simulink model "model"  (Simulink 8.7)
settings: Solver=ode45  StartTime=0.0  StopTime=10.0  FixedStep=Ts  RelTol=1e-3
values from neighbouring files (symbols this model uses):
  Am = 1    [model_params.m]
  NP = 0.001    [model_params.m]
  R = 2    [model_params.m]
  to = round(rand * 100)    [model_params.m]
  Ts = 0.002    [model_params.m]
libraries: commanapbnd3 x2
settings Model: Creator=morozov  LastModifiedBy=morozov
settings DataIOCC: LimitDataPoints=off  SaveFormat=Dataset
settings DebuggingCC: UnderspecifiedInitializationDetection=Simplified  MergeDetectMultiDrivingBlocksExec=error
settings HardwareCC: ProdBitPerPointer=64  ProdLargestAtomicFloat=Float  ProdIntDivRoundTo=Zero  ProdEndianess=LittleEndian  ProdWordSize=64  ProdHWDeviceType=Intel->x86-64 (Windows64)
settings ModelReferenceCC: PropagateSignalLabelsOutOfModel=on
settings ConfigComp: CovModelRefEnable=off

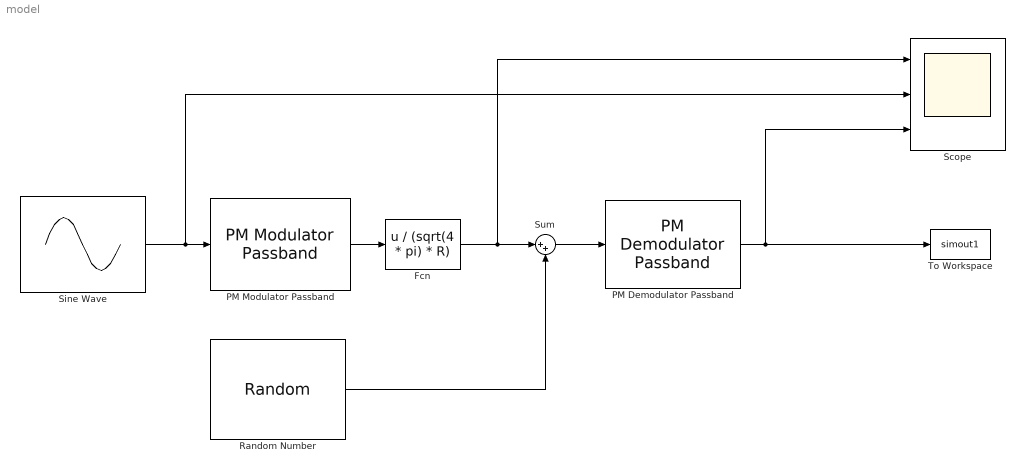
== system model ==
  Fcn : Fcn  Expr=u / (sqrt(4 * pi) * R)
  PM Demodulator Passband : commanapbnd3/PM Demodulator Passband  Fc=carrier_frequency  Ph=0  Kc=pi/2  Ho=100
  PM Modulator Passband : commanapbnd3/PM Modulator Passband  Fc=carrier_frequency  Ph=0  Kc=pi/2
  Random Number : RandomNumber  Variance=NP  Seed=to  SampleTime=Ts
  Scope : Scope  NumInputPorts=3
  Sine Wave : Sin  Amplitude=Am  SampleTime=Ts
  Sum : Sum  Inputs=|++
  To Workspace : ToWorkspace  VariableName=simout1  SampleTime=-1
  wires:
  Sine Wave/1 -> Scope/2, PM Modulator Passband/1
  PM Modulator Passband/1 -> Fcn/1
  PM Demodulator Passband/1 -> To Workspace/1, Scope/3
  Random Number/1 -> Sum/2
  Sum/1 -> PM Demodulator Passband/1
  Fcn/1 -> Scope/1, Sum/1
